simulink model "PI_openloop"  (R2023b)
settings: Solver=ode8  StartTime=0.0  StopTime=20  FixedStep=0.005  RelTol=1e-3
settings Model: Creator=suvo  LastModifiedBy=suvo
settings SolverCC: AlgebraicLoopSolver=TrustRegion
settings DataIOCC: ReturnWorkspaceOutputs=off
settings DebuggingCC: UnconnectedInputMsg=warning  UnconnectedOutputMsg=warning  UnconnectedLineMsg=warning
settings ModelReferenceCC: EnableRefExpFcnMdlSchedulingChecks=on

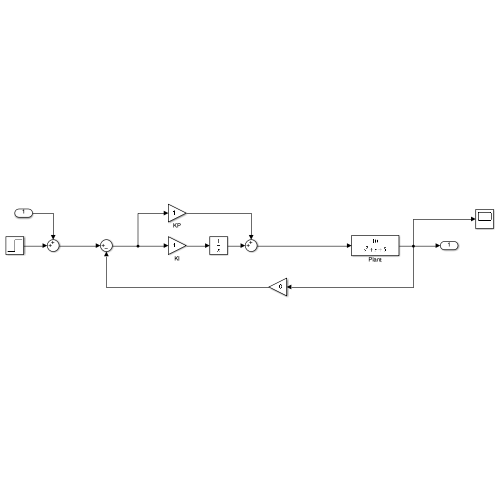
[thumbnail: Simulink's stored preview of the top-level diagram]
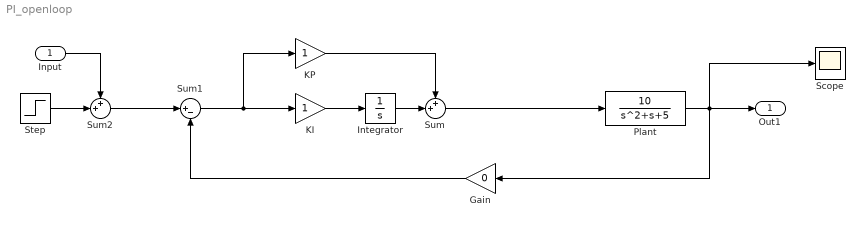
== system PI_openloop ==
  Input : Inport
  Gain : Gain  Gain=0
  Integrator : Integrator
  KI : Gain
  KP : Gain
  Plant : TransferFcn  Numerator=10  Denominator=[1 1 5]
  Scope : Scope
  Step : Step  SampleTime=0
  Sum : Sum  Inputs=++|
  Sum1 : Sum  Inputs=|+-
  Sum2 : Sum  Inputs=++|
  Out1 : Outport
  wires:
  KI/1 -> Integrator/1
  Sum1/1 -> KP/1, KI/1
  KP/1 -> Sum/1
  Integrator/1 -> Sum/2
  Plant/1 -> Out1/1, Gain/1, Scope/1
  Gain/1 -> Sum1/2
  Step/1 -> Sum2/2
  Input/1 -> Sum2/1
  Sum2/1 -> Sum1/1
  Sum/1 -> Plant/1
